simulink model "Actividad2_complemento"  (R2024a)
settings: Solver=VariableStepAuto  StartTime=0.0  StopTime=10.0  MaxStep=0.001  RelTol=1e-3

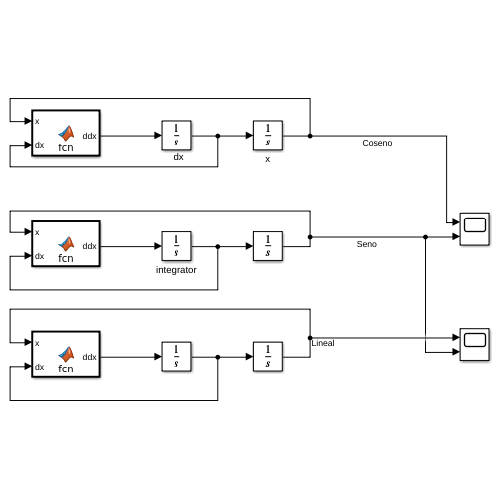
[thumbnail: Simulink's stored preview of the top-level diagram]
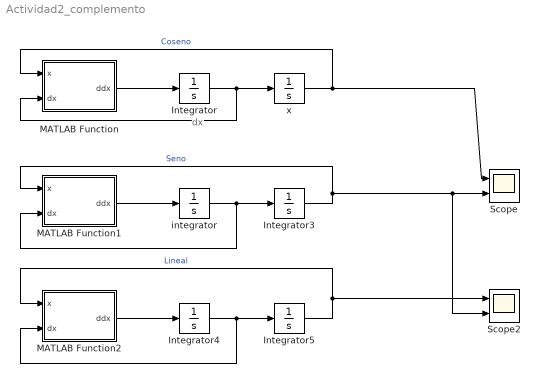
== system Actividad2_complemento ==
  note: dx
  Integrator : Integrator
  Integrator3 : Integrator  InitialCondition=2*pi
  Integrator4 : Integrator
  Integrator5 : Integrator  InitialCondition=2*pi
  MATLAB Function : MATLAB Function  TreatAsAtomicUnit=on
  MATLAB Function1 : MATLAB Function  TreatAsAtomicUnit=on
  MATLAB Function2 : MATLAB Function  TreatAsAtomicUnit=on
  Scope : Scope  NumInputPorts=2
  Scope2 : Scope  NumInputPorts=2
  integrator : Integrator
  x : Integrator  InitialCondition=2*pi
  wires:
  MATLAB Function/1(ddx) -> Integrator/1
  Integrator/1 -> MATLAB Function/2(dx), x/1
  x/1 -> Scope/1, MATLAB Function/1(x)  "Coseno"
  Integrator3/1 -> MATLAB Function1/1(x), Scope2/2, Scope/2  "Seno"
  integrator/1 -> MATLAB Function1/2(dx), Integrator3/1
  MATLAB Function1/1(ddx) -> integrator/1
  Integrator5/1 -> MATLAB Function2/1(x), Scope2/1  "Lineal"
  Integrator4/1 -> MATLAB Function2/2(dx), Integrator5/1
  MATLAB Function2/1(ddx) -> Integrator4/1

== matlab function Actividad2_complemento/MATLAB Function ==
  data: x input; ddx output; dx input
function ddx = fcn(x, dx)
k = 0.5;
m = 0.75;
l = 0.36;
g = 9.8;
Tau= 0.1;
a = l/2;
J=(4*m*a^2)/3;
ddx= Tau/J- k*dx/J- m*g*a*cos(x)/J;

== matlab function Actividad2_complemento/MATLAB Function2 ==
  data: x input; ddx output; dx input
function ddx = fcn(x, dx)
k = 0.5;
m = 0.75;
l = 0.36;
g = 9.8;
Tau= 0.1;
a = l/2;
J=(4*m*a^2)/3;
ddx= Tau/J- k*dx/J- m*g*a*x/J;

== matlab function Actividad2_complemento/MATLAB Function1 ==
  data: x input; ddx output; dx input
function ddx = fcn(x, dx)
k = 0.5;
m = 0.75;
l = 0.36;
g = 9.8;
Tau= 0.1;
a = l/2;
J=(4*m*a^2)/3;
ddx= Tau/J- k*dx/J- m*g*a*sin(x)/J;
